simulink model "Song_Saturation03"  (R2015a)
settings: Solver=ode45  StartTime=0.0  StopTime=90  RelTol=1e-3
undefined symbols (not defined in the file): fdesignblkfcn, gcbh
libraries: dspvision x1, dspsnks4 x1
settings Model: Creator=chulantha  LastModifiedBy=chulantha
settings DebuggingCC: UnderspecifiedInitializationDetection=Classic  MergeDetectMultiDrivingBlocksExec=none  SolverPrmCheckMsg=warning  StateNameClashWarn=warning

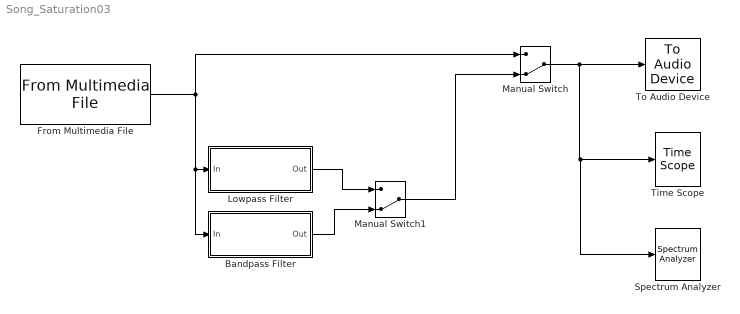
== system Song_Saturation03 ==
  Bandpass Filter : Subsystem  DialogController=fdesignblkfcn  InitFcn=fdesignblkfcn(gcbh, {'InitFcn'});  mask(Bandpass Filter){}
      mask help: Design a bandpass filter
      settings: CopyFcn=fdesignblkfcn(gcbh, {'CopyFcn'});
      mask Help: helpview(mapfilelocation('dsp'), 'dspbandpassfilter');
      mask Display: disp('Bandpass');
  From Multimedia File : dspvision/From Multimedia File  inputFilename=/home/chulantha/Malabe/classes/SignalsAndSystems/Programs/song02.ogg  loop=on  numPlays=inf  outputStreams=Audio only  videoDataType=single  audioDataType=double  inheritSampleTime=on  userDefinedSampleTime=1/30  noAudioOutput=off  isIntensityVideo=off  fourcc=RGB  colorVideoFormat=Separate color signals  outputEOF=off  dataOrg=Column-major  audioFrameSize=1024  computeAudioFrameSize=off  outSamplingMode=Frame based
  Lowpass Filter : Subsystem  DialogController=fdesignblkfcn  InitFcn=fdesignblkfcn(gcbh, {'InitFcn'});  mask(Lowpass Filter){}
      mask help: Design a lowpass filter
      settings: CopyFcn=fdesignblkfcn(gcbh, {'CopyFcn'});
      mask Help: helpview(mapfilelocation('dsp'), 'dsplowpassfilter');
      mask Display: disp('Lowpass')
  Manual Switch : ManualSwitch  CurrentSetting=0
  Manual Switch1 : ManualSwitch  CurrentSetting=0
  Spectrum Analyzer : SpectrumAnalyzer
  Time Scope : TimeScope  DefaultConfigurationName=spbscopes.TimeScopeBlockCfg
  To Audio Device : dspsnks4/To Audio Device  deviceName=Default  inheritSampleRate=on  sampleRate=44100  deviceDatatype=Determine from input data type  autoBufferSize=on  bufferSize=4096  queueDuration=1.0  defaultOutputChannelMapping=on  outputChannelMapping=1:2  outputNumUnderrunSamples=off
  wires:
  Manual Switch/1 -> To Audio Device/1, Spectrum Analyzer/1, Time Scope/1
  From Multimedia File/1 -> Bandpass Filter/1(In), Lowpass Filter/1(In), Manual Switch/1
  Lowpass Filter/1(Out) -> Manual Switch1/1
  Bandpass Filter/1(Out) -> Manual Switch1/2
  Manual Switch1/1 -> Manual Switch/2

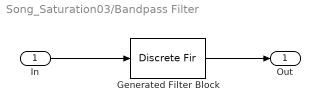
== system Song_Saturation03/Bandpass Filter ==
  In : Inport
  Generated Filter Block : DiscreteFir  Tag=BlockMethodSubSystem  Coefficients=[0.00294564314040180212 0.00799235354356943491 0.012887102654130525 0.0129928113648207118 0.00606740793203454018 -0.00405038713328808187 -0.00897640374660271627 -0.00324534046239173622 0.00853794258633838211 0.0132276001838597546 0.000727053600302059004 -0.0240337891014370808 -0.0420211002462381883 -0.0368793894246286849 -0.0138373928057411513 -0.000627750305474217155 -0.0239940286174276408 -0.0794718146036921674 -0.123680563369359217 -0.102823131717854566 0.00123690806702751038 0.146064387583984268 0.250487192376940282 0.250487192376940282 0.146064387583984268 0.00123690806702751038 -0.102823131717854566 -0.123680563369359217 -0.0794718146036921674 -0.0239940286174276408 -0.000627750305474217155 -0.0138373928057411513 -0.0368793894246286849 -0.0420211002462381883 -0.0240337891014370808 0.000727053600302059004 0.0132276001838597546 0.00853794258633838211 -0.00324534046239173622 -0.00897640374660271627 -0.00405038713328808187 0.00606740793203454018 0.0129928113648207118 0.012887102654130525 0.00799235354356943491 0.00294564314040180212]  InputProcessing=Columns as channels (frame based)
  Out : Outport
  wires:
  In/1 -> Generated Filter Block/1
  Generated Filter Block/1 -> Out/1

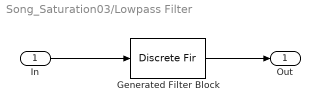
== system Song_Saturation03/Lowpass Filter ==
  In : Inport
  Generated Filter Block : DiscreteFir  Tag=BlockMethodSubSystem  Coefficients=[0.000797645120124761413 0.000956508562077547711 0.00149476014562097722 0.0021985507804132302 0.00308899715795147266 0.0041844687554820556 0.00549876322129311691 0.00704015351359835 0.00880992196535272318 0.0108025989197968499 0.0130040513125740005 0.0153917405781026015 0.0179349073569121491 0.0205941154871042247 0.02332349723883545 0.0260695347766016806 0.0287773811477678582 0.0313854339881610434 0.0338339142268887227 0.0360638961177518896 0.0380184790503336062 0.0396482942005216832 0.0409106198880809721 0.0417715142670424949 0.0422074552299811501 0.0422074552299811501 0.0417715142670424949 0.0409106198880809721 0.0396482942005216832 0.0380184790503336062 0.0360638961177518896 0.0338339142268887227 0.0313854339881610434 0.0287773811477678582 0.0260695347766016806 0.02332349723883545 0.0205941154871042247 0.0179349073569121491 0.0153917405781026015 0.0130040513125740005 0.0108025989197968499 0.00880992196535272318 0.00704015351359835 0.00549876322129311691 0.0041844687554820556 0.00308899715795147266 0.0021985507804132302 0.00149476014562097722 0.000956508562077547711 0.000797645120124761413]  InputProcessing=Columns as channels (frame based)
  Out : Outport
  wires:
  In/1 -> Generated Filter Block/1
  Generated Filter Block/1 -> Out/1
